simulink model "KalmanDados"  (R2021a)
settings: Solver=VariableStepAuto  StartTime=0.0  StopTime=24  RelTol=1e-3
values from neighbouring files (symbols this model uses):
  kalmfpitch = kalmfpitch(1,:)    [parse3e4_kalmanSemBias.m]
  kalmfroll = kalmfroll(1,:)    [parse3e4_kalmanSemBias.m]
settings Model: Creator=Pedrus  LastModifiedBy=Pedrus

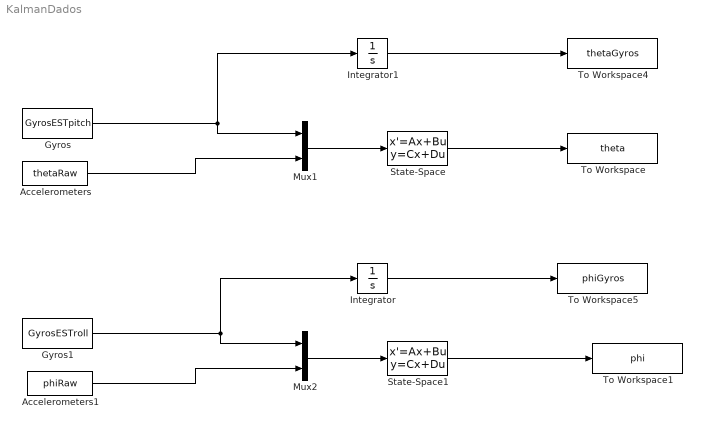
== system KalmanDados ==
  Accelerometers : FromWorkspace  VariableName=thetaRaw
  Accelerometers1 : FromWorkspace  VariableName=phiRaw
  Gyros : FromWorkspace  VariableName=GyrosESTpitch
  Gyros1 : FromWorkspace  VariableName=GyrosESTroll
  Integrator : Integrator
  Integrator1 : Integrator
  Mux1 : Mux  Inputs=2
  Mux2 : Mux  Inputs=2
  State-Space : StateSpace  A=kalmfpitch.A  B=kalmfpitch.B  C=kalmfpitch.C  D=kalmfpitch.D  InitialCondition=0
  State-Space1 : StateSpace  A=kalmfroll.A  B=kalmfroll.B  C=kalmfroll.C  D=kalmfroll.D  InitialCondition=0
  To Workspace : ToWorkspace  VariableName=theta  SaveFormat=Timeseries  SampleTime=-1
  To Workspace1 : ToWorkspace  VariableName=phi  SaveFormat=Timeseries  SampleTime=-1
  To Workspace4 : ToWorkspace  VariableName=thetaGyros  SaveFormat=Timeseries  SampleTime=-1
  To Workspace5 : ToWorkspace  VariableName=phiGyros  SaveFormat=Timeseries  SampleTime=-1
  wires:
  Integrator1/1 -> To Workspace4/1
  Integrator/1 -> To Workspace5/1
  Gyros/1 -> Mux1/1, Integrator1/1
  Mux1/1 -> State-Space/1
  State-Space/1 -> To Workspace/1
  Accelerometers/1 -> Mux1/2
  Accelerometers1/1 -> Mux2/2
  Mux2/1 -> State-Space1/1
  Gyros1/1 -> Mux2/1, Integrator/1
  State-Space1/1 -> To Workspace1/1
